simulink model "G_cl_PA"  (R2020b)
settings: Solver=VariableStepAuto  StartTime=0.0  StopTime=10.0  RelTol=1e-3
libraries: fod x1, cstblocks x1
settings Model: Creator=jasper  LastModifiedBy=jasper

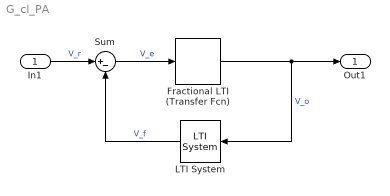
== system G_cl_PA ==
  In1 : Inport
  Fractional LTI (Transfer Fcn) : fod/Fractional LTI (Transfer Fcn)  G=A_PA  freqRange=[0.001 1000]  approxNum=5  useRef=off
      settings: SourceProductName=FOMCON Toolbox
  LTI System : cstblocks/LTI System  sys=f  IC=[]
  Sum : Sum  Inputs=|+-
  Out1 : Outport  SignalName=V_o
  wires:
  Sum/1 -> Fractional LTI (Transfer Fcn)/1  "V_e"
  LTI System/1 -> Sum/2  "V_f"
  Fractional LTI (Transfer Fcn)/1 -> Out1/1, LTI System/1  "V_o"
  In1/1 -> Sum/1  "V_r"
